simulink model "Digital-Memory-Architecture"  (R2024b)
settings: Solver=VariableStepAuto  StartTime=0.0  StopTime=10.0  RelTol=1e-3
libraries: simulink_extras x129
(part 2 of 5)

== system Digital-Memory-Architecture/8to1MUX7 ==
  Adress0 : Inport
  Adress1 : Inport  Port=2
  Adress2 : Inport  Port=3
  D0 : Inport  Port=4
  D1 : Inport  Port=5
  D2 : Inport  Port=6
  D3 : Inport  Port=7
  D4 : Inport  Port=8
  D5 : Inport  Port=9
  D6 : Inport  Port=10
  D7 : Inport  Port=11
  Logical Operator : Logic  Operator=NOT  IconShape=distinctive  AllPortsSameDT=off  OutDataTypeStr=boolean
  Logical Operator1 : Logic  Operator=NOT  IconShape=distinctive  AllPortsSameDT=off  OutDataTypeStr=boolean
  Logical Operator{4..11} (8 alike) : Logic  Inputs=4  IconShape=distinctive  AllPortsSameDT=off  OutDataTypeStr=boolean
  Logical Operator2 : Logic  Operator=NOT  IconShape=distinctive  AllPortsSameDT=off  OutDataTypeStr=boolean
  Logical Operator3 : Logic  Operator=OR  Inputs=8  IconShape=distinctive  AllPortsSameDT=off  OutDataTypeStr=boolean
  D : Outport
  wires:
  Logical Operator3/1 -> D/1
  Adress0/1 -> Logical Operator11/1, Logical Operator9/1, Logical Operator7/1, Logical Operator5/1, Logical Operator/1
  Adress1/1 -> Logical Operator11/2, Logical Operator10/2, Logical Operator7/2, Logical Operator6/2, Logical Operator1/1
  Adress2/1 -> Logical Operator11/3, Logical Operator10/3, Logical Operator9/3, Logical Operator8/3, Logical Operator2/1
  D7/1 -> Logical Operator11/4
  D6/1 -> Logical Operator10/4
  D5/1 -> Logical Operator9/4
  D4/1 -> Logical Operator8/4
  D3/1 -> Logical Operator7/4
  D2/1 -> Logical Operator6/4
  D1/1 -> Logical Operator5/4
  D0/1 -> Logical Operator4/4
  Logical Operator2/1 -> Logical Operator7/3, Logical Operator6/3, Logical Operator5/3, Logical Operator4/3
  Logical Operator1/1 -> Logical Operator9/2, Logical Operator8/2, Logical Operator5/2, Logical Operator4/2
  Logical Operator/1 -> Logical Operator10/1, Logical Operator8/1, Logical Operator6/1, Logical Operator4/1
  Logical Operator4/1 -> Logical Operator3/1
  Logical Operator5/1 -> Logical Operator3/2
  Logical Operator6/1 -> Logical Operator3/3
  Logical Operator7/1 -> Logical Operator3/4
  Logical Operator8/1 -> Logical Operator3/5
  Logical Operator9/1 -> Logical Operator3/6
  Logical Operator10/1 -> Logical Operator3/7
  Logical Operator11/1 -> Logical Operator3/8

== system Digital-Memory-Architecture/8to1MUX8 ==
  Adress0 : Inport
  Adress1 : Inport  Port=2
  Adress2 : Inport  Port=3
  D0 : Inport  Port=4
  D1 : Inport  Port=5
  D2 : Inport  Port=6
  D3 : Inport  Port=7
  D4 : Inport  Port=8
  D5 : Inport  Port=9
  D6 : Inport  Port=10
  D7 : Inport  Port=11
  Logical Operator : Logic  Operator=NOT  IconShape=distinctive  AllPortsSameDT=off  OutDataTypeStr=boolean
  Logical Operator1 : Logic  Operator=NOT  IconShape=distinctive  AllPortsSameDT=off  OutDataTypeStr=boolean
  Logical Operator{4..11} (8 alike) : Logic  Inputs=4  IconShape=distinctive  AllPortsSameDT=off  OutDataTypeStr=boolean
  Logical Operator2 : Logic  Operator=NOT  IconShape=distinctive  AllPortsSameDT=off  OutDataTypeStr=boolean
  Logical Operator3 : Logic  Operator=OR  Inputs=8  IconShape=distinctive  AllPortsSameDT=off  OutDataTypeStr=boolean
  A : Outport
  wires:
  Logical Operator3/1 -> A/1
  Adress0/1 -> Logical Operator11/1, Logical Operator9/1, Logical Operator7/1, Logical Operator5/1, Logical Operator/1
  Adress1/1 -> Logical Operator11/2, Logical Operator10/2, Logical Operator7/2, Logical Operator6/2, Logical Operator1/1
  Adress2/1 -> Logical Operator11/3, Logical Operator10/3, Logical Operator9/3, Logical Operator8/3, Logical Operator2/1
  D7/1 -> Logical Operator11/4
  D6/1 -> Logical Operator10/4
  D5/1 -> Logical Operator9/4
  D4/1 -> Logical Operator8/4
  D3/1 -> Logical Operator7/4
  D2/1 -> Logical Operator6/4
  D1/1 -> Logical Operator5/4
  D0/1 -> Logical Operator4/4
  Logical Operator2/1 -> Logical Operator7/3, Logical Operator6/3, Logical Operator5/3, Logical Operator4/3
  Logical Operator1/1 -> Logical Operator9/2, Logical Operator8/2, Logical Operator5/2, Logical Operator4/2
  Logical Operator/1 -> Logical Operator10/1, Logical Operator8/1, Logical Operator6/1, Logical Operator4/1
  Logical Operator4/1 -> Logical Operator3/1
  Logical Operator5/1 -> Logical Operator3/2
  Logical Operator6/1 -> Logical Operator3/3
  Logical Operator7/1 -> Logical Operator3/4
  Logical Operator8/1 -> Logical Operator3/5
  Logical Operator9/1 -> Logical Operator3/6
  Logical Operator10/1 -> Logical Operator3/7
  Logical Operator11/1 -> Logical Operator3/8

== system Digital-Memory-Architecture/8to1MUX9 ==
  Adress0 : Inport
  Adress1 : Inport  Port=2
  Adress2 : Inport  Port=3
  D0 : Inport  Port=4
  D1 : Inport  Port=5
  D2 : Inport  Port=6
  D3 : Inport  Port=7
  D4 : Inport  Port=8
  D5 : Inport  Port=9
  D6 : Inport  Port=10
  D7 : Inport  Port=11
  Logical Operator : Logic  Operator=NOT  IconShape=distinctive  AllPortsSameDT=off  OutDataTypeStr=boolean
  Logical Operator1 : Logic  Operator=NOT  IconShape=distinctive  AllPortsSameDT=off  OutDataTypeStr=boolean
  Logical Operator{4..11} (8 alike) : Logic  Inputs=4  IconShape=distinctive  AllPortsSameDT=off  OutDataTypeStr=boolean
  Logical Operator2 : Logic  Operator=NOT  IconShape=distinctive  AllPortsSameDT=off  OutDataTypeStr=boolean
  Logical Operator3 : Logic  Operator=OR  Inputs=8  IconShape=distinctive  AllPortsSameDT=off  OutDataTypeStr=boolean
  B : Outport
  wires:
  Logical Operator3/1 -> B/1
  Adress0/1 -> Logical Operator11/1, Logical Operator9/1, Logical Operator7/1, Logical Operator5/1, Logical Operator/1
  Adress1/1 -> Logical Operator11/2, Logical Operator10/2, Logical Operator7/2, Logical Operator6/2, Logical Operator1/1
  Adress2/1 -> Logical Operator11/3, Logical Operator10/3, Logical Operator9/3, Logical Operator8/3, Logical Operator2/1
  D7/1 -> Logical Operator11/4
  D6/1 -> Logical Operator10/4
  D5/1 -> Logical Operator9/4
  D4/1 -> Logical Operator8/4
  D3/1 -> Logical Operator7/4
  D2/1 -> Logical Operator6/4
  D1/1 -> Logical Operator5/4
  D0/1 -> Logical Operator4/4
  Logical Operator2/1 -> Logical Operator7/3, Logical Operator6/3, Logical Operator5/3, Logical Operator4/3
  Logical Operator1/1 -> Logical Operator9/2, Logical Operator8/2, Logical Operator5/2, Logical Operator4/2
  Logical Operator/1 -> Logical Operator10/1, Logical Operator8/1, Logical Operator6/1, Logical Operator4/1
  Logical Operator4/1 -> Logical Operator3/1
  Logical Operator5/1 -> Logical Operator3/2
  Logical Operator6/1 -> Logical Operator3/3
  Logical Operator7/1 -> Logical Operator3/4
  Logical Operator8/1 -> Logical Operator3/5
  Logical Operator9/1 -> Logical Operator3/6
  Logical Operator10/1 -> Logical Operator3/7
  Logical Operator11/1 -> Logical Operator3/8

== system Digital-Memory-Architecture/BitCell1 ==
  D : Inport
  WE : Inport  Port=2
  CLK : Inport  Port=3
  Constant : Constant
  D Flip-Flop : simulink_extras/Flip Flops/D Flip-Flop
  Logical Operator : Logic  Operator=NOT  IconShape=distinctive  AllPortsSameDT=off  OutDataTypeStr=boolean
  Logical Operator1 : Logic  IconShape=distinctive  AllPortsSameDT=off  OutDataTypeStr=boolean
  Logical Operator2 : Logic  IconShape=distinctive  AllPortsSameDT=off  OutDataTypeStr=boolean
  Logical Operator3 : Logic  Operator=OR  IconShape=distinctive  AllPortsSameDT=off  OutDataTypeStr=boolean
  Q : Outport
  wires:
  Logical Operator2/1 -> Logical Operator3/2
  CLK/1 -> D Flip-Flop/2
  Logical Operator1/1 -> Logical Operator3/1
  Constant/1 -> D Flip-Flop/3
  D Flip-Flop/1 -> Q/1, Logical Operator2/2
  Logical Operator3/1 -> D Flip-Flop/1
  Logical Operator/1 -> Logical Operator2/1
  WE/1 -> Logical Operator/1, Logical Operator1/2
  D/1 -> Logical Operator1/1

== system Digital-Memory-Architecture/BitCell10 ==
  D : Inport
  WE : Inport  Port=2
  CLK : Inport  Port=3
  Constant : Constant
  D Flip-Flop : simulink_extras/Flip Flops/D Flip-Flop
  Logical Operator : Logic  Operator=NOT  IconShape=distinctive  AllPortsSameDT=off  OutDataTypeStr=boolean
  Logical Operator1 : Logic  IconShape=distinctive  AllPortsSameDT=off  OutDataTypeStr=boolean
  Logical Operator2 : Logic  IconShape=distinctive  AllPortsSameDT=off  OutDataTypeStr=boolean
  Logical Operator3 : Logic  Operator=OR  IconShape=distinctive  AllPortsSameDT=off  OutDataTypeStr=boolean
  Q : Outport
  wires:
  Logical Operator2/1 -> Logical Operator3/2
  CLK/1 -> D Flip-Flop/2
  Logical Operator1/1 -> Logical Operator3/1
  Constant/1 -> D Flip-Flop/3
  D Flip-Flop/1 -> Q/1, Logical Operator2/2
  Logical Operator3/1 -> D Flip-Flop/1
  Logical Operator/1 -> Logical Operator2/1
  WE/1 -> Logical Operator/1, Logical Operator1/2
  D/1 -> Logical Operator1/1

== system Digital-Memory-Architecture/BitCell100 ==
  D : Inport
  WE : Inport  Port=2
  CLK : Inport  Port=3
  Constant : Constant
  D Flip-Flop : simulink_extras/Flip Flops/D Flip-Flop
  Logical Operator : Logic  Operator=NOT  IconShape=distinctive  AllPortsSameDT=off  OutDataTypeStr=boolean
  Logical Operator1 : Logic  IconShape=distinctive  AllPortsSameDT=off  OutDataTypeStr=boolean
  Logical Operator2 : Logic  IconShape=distinctive  AllPortsSameDT=off  OutDataTypeStr=boolean
  Logical Operator3 : Logic  Operator=OR  IconShape=distinctive  AllPortsSameDT=off  OutDataTypeStr=boolean
  Q : Outport
  wires:
  Logical Operator2/1 -> Logical Operator3/2
  CLK/1 -> D Flip-Flop/2
  Logical Operator1/1 -> Logical Operator3/1
  Constant/1 -> D Flip-Flop/3
  D Flip-Flop/1 -> Q/1, Logical Operator2/2
  Logical Operator3/1 -> D Flip-Flop/1
  Logical Operator/1 -> Logical Operator2/1
  WE/1 -> Logical Operator/1, Logical Operator1/2
  D/1 -> Logical Operator1/1

== system Digital-Memory-Architecture/BitCell101 ==
  D : Inport
  WE : Inport  Port=2
  CLK : Inport  Port=3
  Constant : Constant
  D Flip-Flop : simulink_extras/Flip Flops/D Flip-Flop
  Logical Operator : Logic  Operator=NOT  IconShape=distinctive  AllPortsSameDT=off  OutDataTypeStr=boolean
  Logical Operator1 : Logic  IconShape=distinctive  AllPortsSameDT=off  OutDataTypeStr=boolean
  Logical Operator2 : Logic  IconShape=distinctive  AllPortsSameDT=off  OutDataTypeStr=boolean
  Logical Operator3 : Logic  Operator=OR  IconShape=distinctive  AllPortsSameDT=off  OutDataTypeStr=boolean
  Q : Outport
  wires:
  Logical Operator2/1 -> Logical Operator3/2
  CLK/1 -> D Flip-Flop/2
  Logical Operator1/1 -> Logical Operator3/1
  Constant/1 -> D Flip-Flop/3
  D Flip-Flop/1 -> Q/1, Logical Operator2/2
  Logical Operator3/1 -> D Flip-Flop/1
  Logical Operator/1 -> Logical Operator2/1
  WE/1 -> Logical Operator/1, Logical Operator1/2
  D/1 -> Logical Operator1/1

== system Digital-Memory-Architecture/BitCell102 ==
  D : Inport
  WE : Inport  Port=2
  CLK : Inport  Port=3
  Constant : Constant
  D Flip-Flop : simulink_extras/Flip Flops/D Flip-Flop
  Logical Operator : Logic  Operator=NOT  IconShape=distinctive  AllPortsSameDT=off  OutDataTypeStr=boolean
  Logical Operator1 : Logic  IconShape=distinctive  AllPortsSameDT=off  OutDataTypeStr=boolean
  Logical Operator2 : Logic  IconShape=distinctive  AllPortsSameDT=off  OutDataTypeStr=boolean
  Logical Operator3 : Logic  Operator=OR  IconShape=distinctive  AllPortsSameDT=off  OutDataTypeStr=boolean
  Q : Outport
  wires:
  Logical Operator2/1 -> Logical Operator3/2
  CLK/1 -> D Flip-Flop/2
  Logical Operator1/1 -> Logical Operator3/1
  Constant/1 -> D Flip-Flop/3
  D Flip-Flop/1 -> Q/1, Logical Operator2/2
  Logical Operator3/1 -> D Flip-Flop/1
  Logical Operator/1 -> Logical Operator2/1
  WE/1 -> Logical Operator/1, Logical Operator1/2
  D/1 -> Logical Operator1/1

== system Digital-Memory-Architecture/BitCell103 ==
  D : Inport
  WE : Inport  Port=2
  CLK : Inport  Port=3
  Constant : Constant
  D Flip-Flop : simulink_extras/Flip Flops/D Flip-Flop
  Logical Operator : Logic  Operator=NOT  IconShape=distinctive  AllPortsSameDT=off  OutDataTypeStr=boolean
  Logical Operator1 : Logic  IconShape=distinctive  AllPortsSameDT=off  OutDataTypeStr=boolean
  Logical Operator2 : Logic  IconShape=distinctive  AllPortsSameDT=off  OutDataTypeStr=boolean
  Logical Operator3 : Logic  Operator=OR  IconShape=distinctive  AllPortsSameDT=off  OutDataTypeStr=boolean
  Q : Outport
  wires:
  Logical Operator2/1 -> Logical Operator3/2
  CLK/1 -> D Flip-Flop/2
  Logical Operator1/1 -> Logical Operator3/1
  Constant/1 -> D Flip-Flop/3
  D Flip-Flop/1 -> Q/1, Logical Operator2/2
  Logical Operator3/1 -> D Flip-Flop/1
  Logical Operator/1 -> Logical Operator2/1
  WE/1 -> Logical Operator/1, Logical Operator1/2
  D/1 -> Logical Operator1/1

== system Digital-Memory-Architecture/BitCell104 ==
  D : Inport
  WE : Inport  Port=2
  CLK : Inport  Port=3
  Constant : Constant
  D Flip-Flop : simulink_extras/Flip Flops/D Flip-Flop
  Logical Operator : Logic  Operator=NOT  IconShape=distinctive  AllPortsSameDT=off  OutDataTypeStr=boolean
  Logical Operator1 : Logic  IconShape=distinctive  AllPortsSameDT=off  OutDataTypeStr=boolean
  Logical Operator2 : Logic  IconShape=distinctive  AllPortsSameDT=off  OutDataTypeStr=boolean
  Logical Operator3 : Logic  Operator=OR  IconShape=distinctive  AllPortsSameDT=off  OutDataTypeStr=boolean
  Q : Outport
  wires:
  Logical Operator2/1 -> Logical Operator3/2
  CLK/1 -> D Flip-Flop/2
  Logical Operator1/1 -> Logical Operator3/1
  Constant/1 -> D Flip-Flop/3
  D Flip-Flop/1 -> Q/1, Logical Operator2/2
  Logical Operator3/1 -> D Flip-Flop/1
  Logical Operator/1 -> Logical Operator2/1
  WE/1 -> Logical Operator/1, Logical Operator1/2
  D/1 -> Logical Operator1/1

== system Digital-Memory-Architecture/BitCell105 ==
  D : Inport
  WE : Inport  Port=2
  CLK : Inport  Port=3
  Constant : Constant
  D Flip-Flop : simulink_extras/Flip Flops/D Flip-Flop
  Logical Operator : Logic  Operator=NOT  IconShape=distinctive  AllPortsSameDT=off  OutDataTypeStr=boolean
  Logical Operator1 : Logic  IconShape=distinctive  AllPortsSameDT=off  OutDataTypeStr=boolean
  Logical Operator2 : Logic  IconShape=distinctive  AllPortsSameDT=off  OutDataTypeStr=boolean
  Logical Operator3 : Logic  Operator=OR  IconShape=distinctive  AllPortsSameDT=off  OutDataTypeStr=boolean
  Q : Outport
  wires:
  Logical Operator2/1 -> Logical Operator3/2
  CLK/1 -> D Flip-Flop/2
  Logical Operator1/1 -> Logical Operator3/1
  Constant/1 -> D Flip-Flop/3
  D Flip-Flop/1 -> Q/1, Logical Operator2/2
  Logical Operator3/1 -> D Flip-Flop/1
  Logical Operator/1 -> Logical Operator2/1
  WE/1 -> Logical Operator/1, Logical Operator1/2
  D/1 -> Logical Operator1/1

== system Digital-Memory-Architecture/BitCell106 ==
  D : Inport
  WE : Inport  Port=2
  CLK : Inport  Port=3
  Constant : Constant
  D Flip-Flop : simulink_extras/Flip Flops/D Flip-Flop
  Logical Operator : Logic  Operator=NOT  IconShape=distinctive  AllPortsSameDT=off  OutDataTypeStr=boolean
  Logical Operator1 : Logic  IconShape=distinctive  AllPortsSameDT=off  OutDataTypeStr=boolean
  Logical Operator2 : Logic  IconShape=distinctive  AllPortsSameDT=off  OutDataTypeStr=boolean
  Logical Operator3 : Logic  Operator=OR  IconShape=distinctive  AllPortsSameDT=off  OutDataTypeStr=boolean
  Q : Outport
  wires:
  Logical Operator2/1 -> Logical Operator3/2
  CLK/1 -> D Flip-Flop/2
  Logical Operator1/1 -> Logical Operator3/1
  Constant/1 -> D Flip-Flop/3
  D Flip-Flop/1 -> Q/1, Logical Operator2/2
  Logical Operator3/1 -> D Flip-Flop/1
  Logical Operator/1 -> Logical Operator2/1
  WE/1 -> Logical Operator/1, Logical Operator1/2
  D/1 -> Logical Operator1/1

== system Digital-Memory-Architecture/BitCell107 ==
  D : Inport
  WE : Inport  Port=2
  CLK : Inport  Port=3
  Constant : Constant
  D Flip-Flop : simulink_extras/Flip Flops/D Flip-Flop
  Logical Operator : Logic  Operator=NOT  IconShape=distinctive  AllPortsSameDT=off  OutDataTypeStr=boolean
  Logical Operator1 : Logic  IconShape=distinctive  AllPortsSameDT=off  OutDataTypeStr=boolean
  Logical Operator2 : Logic  IconShape=distinctive  AllPortsSameDT=off  OutDataTypeStr=boolean
  Logical Operator3 : Logic  Operator=OR  IconShape=distinctive  AllPortsSameDT=off  OutDataTypeStr=boolean
  Q : Outport
  wires:
  Logical Operator2/1 -> Logical Operator3/2
  CLK/1 -> D Flip-Flop/2
  Logical Operator1/1 -> Logical Operator3/1
  Constant/1 -> D Flip-Flop/3
  D Flip-Flop/1 -> Q/1, Logical Operator2/2
  Logical Operator3/1 -> D Flip-Flop/1
  Logical Operator/1 -> Logical Operator2/1
  WE/1 -> Logical Operator/1, Logical Operator1/2
  D/1 -> Logical Operator1/1

== system Digital-Memory-Architecture/BitCell108 ==
  D : Inport
  WE : Inport  Port=2
  CLK : Inport  Port=3
  Constant : Constant
  D Flip-Flop : simulink_extras/Flip Flops/D Flip-Flop
  Logical Operator : Logic  Operator=NOT  IconShape=distinctive  AllPortsSameDT=off  OutDataTypeStr=boolean
  Logical Operator1 : Logic  IconShape=distinctive  AllPortsSameDT=off  OutDataTypeStr=boolean
  Logical Operator2 : Logic  IconShape=distinctive  AllPortsSameDT=off  OutDataTypeStr=boolean
  Logical Operator3 : Logic  Operator=OR  IconShape=distinctive  AllPortsSameDT=off  OutDataTypeStr=boolean
  Q : Outport
  wires:
  Logical Operator2/1 -> Logical Operator3/2
  CLK/1 -> D Flip-Flop/2
  Logical Operator1/1 -> Logical Operator3/1
  Constant/1 -> D Flip-Flop/3
  D Flip-Flop/1 -> Q/1, Logical Operator2/2
  Logical Operator3/1 -> D Flip-Flop/1
  Logical Operator/1 -> Logical Operator2/1
  WE/1 -> Logical Operator/1, Logical Operator1/2
  D/1 -> Logical Operator1/1

== system Digital-Memory-Architecture/BitCell109 ==
  D : Inport
  WE : Inport  Port=2
  CLK : Inport  Port=3
  Constant : Constant
  D Flip-Flop : simulink_extras/Flip Flops/D Flip-Flop
  Logical Operator : Logic  Operator=NOT  IconShape=distinctive  AllPortsSameDT=off  OutDataTypeStr=boolean
  Logical Operator1 : Logic  IconShape=distinctive  AllPortsSameDT=off  OutDataTypeStr=boolean
  Logical Operator2 : Logic  IconShape=distinctive  AllPortsSameDT=off  OutDataTypeStr=boolean
  Logical Operator3 : Logic  Operator=OR  IconShape=distinctive  AllPortsSameDT=off  OutDataTypeStr=boolean
  Q : Outport
  wires:
  Logical Operator2/1 -> Logical Operator3/2
  CLK/1 -> D Flip-Flop/2
  Logical Operator1/1 -> Logical Operator3/1
  Constant/1 -> D Flip-Flop/3
  D Flip-Flop/1 -> Q/1, Logical Operator2/2
  Logical Operator3/1 -> D Flip-Flop/1
  Logical Operator/1 -> Logical Operator2/1
  WE/1 -> Logical Operator/1, Logical Operator1/2
  D/1 -> Logical Operator1/1

== system Digital-Memory-Architecture/BitCell11 ==
  D : Inport
  WE : Inport  Port=2
  CLK : Inport  Port=3
  Constant : Constant
  D Flip-Flop : simulink_extras/Flip Flops/D Flip-Flop
  Logical Operator : Logic  Operator=NOT  IconShape=distinctive  AllPortsSameDT=off  OutDataTypeStr=boolean
  Logical Operator1 : Logic  IconShape=distinctive  AllPortsSameDT=off  OutDataTypeStr=boolean
  Logical Operator2 : Logic  IconShape=distinctive  AllPortsSameDT=off  OutDataTypeStr=boolean
  Logical Operator3 : Logic  Operator=OR  IconShape=distinctive  AllPortsSameDT=off  OutDataTypeStr=boolean
  Q : Outport
  wires:
  Logical Operator2/1 -> Logical Operator3/2
  CLK/1 -> D Flip-Flop/2
  Logical Operator1/1 -> Logical Operator3/1
  Constant/1 -> D Flip-Flop/3
  D Flip-Flop/1 -> Q/1, Logical Operator2/2
  Logical Operator3/1 -> D Flip-Flop/1
  Logical Operator/1 -> Logical Operator2/1
  WE/1 -> Logical Operator/1, Logical Operator1/2
  D/1 -> Logical Operator1/1

== system Digital-Memory-Architecture/BitCell110 ==
  D : Inport
  WE : Inport  Port=2
  CLK : Inport  Port=3
  Constant : Constant
  D Flip-Flop : simulink_extras/Flip Flops/D Flip-Flop
  Logical Operator : Logic  Operator=NOT  IconShape=distinctive  AllPortsSameDT=off  OutDataTypeStr=boolean
  Logical Operator1 : Logic  IconShape=distinctive  AllPortsSameDT=off  OutDataTypeStr=boolean
  Logical Operator2 : Logic  IconShape=distinctive  AllPortsSameDT=off  OutDataTypeStr=boolean
  Logical Operator3 : Logic  Operator=OR  IconShape=distinctive  AllPortsSameDT=off  OutDataTypeStr=boolean
  Q : Outport
  wires:
  Logical Operator2/1 -> Logical Operator3/2
  CLK/1 -> D Flip-Flop/2
  Logical Operator1/1 -> Logical Operator3/1
  Constant/1 -> D Flip-Flop/3
  D Flip-Flop/1 -> Q/1, Logical Operator2/2
  Logical Operator3/1 -> D Flip-Flop/1
  Logical Operator/1 -> Logical Operator2/1
  WE/1 -> Logical Operator/1, Logical Operator1/2
  D/1 -> Logical Operator1/1

== system Digital-Memory-Architecture/BitCell111 ==
  D : Inport
  WE : Inport  Port=2
  CLK : Inport  Port=3
  Constant : Constant
  D Flip-Flop : simulink_extras/Flip Flops/D Flip-Flop
  Logical Operator : Logic  Operator=NOT  IconShape=distinctive  AllPortsSameDT=off  OutDataTypeStr=boolean
  Logical Operator1 : Logic  IconShape=distinctive  AllPortsSameDT=off  OutDataTypeStr=boolean
  Logical Operator2 : Logic  IconShape=distinctive  AllPortsSameDT=off  OutDataTypeStr=boolean
  Logical Operator3 : Logic  Operator=OR  IconShape=distinctive  AllPortsSameDT=off  OutDataTypeStr=boolean
  Q : Outport
  wires:
  Logical Operator2/1 -> Logical Operator3/2
  CLK/1 -> D Flip-Flop/2
  Logical Operator1/1 -> Logical Operator3/1
  Constant/1 -> D Flip-Flop/3
  D Flip-Flop/1 -> Q/1, Logical Operator2/2
  Logical Operator3/1 -> D Flip-Flop/1
  Logical Operator/1 -> Logical Operator2/1
  WE/1 -> Logical Operator/1, Logical Operator1/2
  D/1 -> Logical Operator1/1

== system Digital-Memory-Architecture/BitCell112 ==
  D : Inport
  WE : Inport  Port=2
  CLK : Inport  Port=3
  Constant : Constant
  D Flip-Flop : simulink_extras/Flip Flops/D Flip-Flop
  Logical Operator : Logic  Operator=NOT  IconShape=distinctive  AllPortsSameDT=off  OutDataTypeStr=boolean
  Logical Operator1 : Logic  IconShape=distinctive  AllPortsSameDT=off  OutDataTypeStr=boolean
  Logical Operator2 : Logic  IconShape=distinctive  AllPortsSameDT=off  OutDataTypeStr=boolean
  Logical Operator3 : Logic  Operator=OR  IconShape=distinctive  AllPortsSameDT=off  OutDataTypeStr=boolean
  Q : Outport
  wires:
  Logical Operator2/1 -> Logical Operator3/2
  CLK/1 -> D Flip-Flop/2
  Logical Operator1/1 -> Logical Operator3/1
  Constant/1 -> D Flip-Flop/3
  D Flip-Flop/1 -> Q/1, Logical Operator2/2
  Logical Operator3/1 -> D Flip-Flop/1
  Logical Operator/1 -> Logical Operator2/1
  WE/1 -> Logical Operator/1, Logical Operator1/2
  D/1 -> Logical Operator1/1

== system Digital-Memory-Architecture/BitCell113 ==
  D : Inport
  WE : Inport  Port=2
  CLK : Inport  Port=3
  Constant : Constant
  D Flip-Flop : simulink_extras/Flip Flops/D Flip-Flop
  Logical Operator : Logic  Operator=NOT  IconShape=distinctive  AllPortsSameDT=off  OutDataTypeStr=boolean
  Logical Operator1 : Logic  IconShape=distinctive  AllPortsSameDT=off  OutDataTypeStr=boolean
  Logical Operator2 : Logic  IconShape=distinctive  AllPortsSameDT=off  OutDataTypeStr=boolean
  Logical Operator3 : Logic  Operator=OR  IconShape=distinctive  AllPortsSameDT=off  OutDataTypeStr=boolean
  Q : Outport
  wires:
  Logical Operator2/1 -> Logical Operator3/2
  CLK/1 -> D Flip-Flop/2
  Logical Operator1/1 -> Logical Operator3/1
  Constant/1 -> D Flip-Flop/3
  D Flip-Flop/1 -> Q/1, Logical Operator2/2
  Logical Operator3/1 -> D Flip-Flop/1
  Logical Operator/1 -> Logical Operator2/1
  WE/1 -> Logical Operator/1, Logical Operator1/2
  D/1 -> Logical Operator1/1

== system Digital-Memory-Architecture/BitCell114 ==
  D : Inport
  WE : Inport  Port=2
  CLK : Inport  Port=3
  Constant : Constant
  D Flip-Flop : simulink_extras/Flip Flops/D Flip-Flop
  Logical Operator : Logic  Operator=NOT  IconShape=distinctive  AllPortsSameDT=off  OutDataTypeStr=boolean
  Logical Operator1 : Logic  IconShape=distinctive  AllPortsSameDT=off  OutDataTypeStr=boolean
  Logical Operator2 : Logic  IconShape=distinctive  AllPortsSameDT=off  OutDataTypeStr=boolean
  Logical Operator3 : Logic  Operator=OR  IconShape=distinctive  AllPortsSameDT=off  OutDataTypeStr=boolean
  Q : Outport
  wires:
  Logical Operator2/1 -> Logical Operator3/2
  CLK/1 -> D Flip-Flop/2
  Logical Operator1/1 -> Logical Operator3/1
  Constant/1 -> D Flip-Flop/3
  D Flip-Flop/1 -> Q/1, Logical Operator2/2
  Logical Operator3/1 -> D Flip-Flop/1
  Logical Operator/1 -> Logical Operator2/1
  WE/1 -> Logical Operator/1, Logical Operator1/2
  D/1 -> Logical Operator1/1

== system Digital-Memory-Architecture/BitCell115 ==
  D : Inport
  WE : Inport  Port=2
  CLK : Inport  Port=3
  Constant : Constant
  D Flip-Flop : simulink_extras/Flip Flops/D Flip-Flop
  Logical Operator : Logic  Operator=NOT  IconShape=distinctive  AllPortsSameDT=off  OutDataTypeStr=boolean
  Logical Operator1 : Logic  IconShape=distinctive  AllPortsSameDT=off  OutDataTypeStr=boolean
  Logical Operator2 : Logic  IconShape=distinctive  AllPortsSameDT=off  OutDataTypeStr=boolean
  Logical Operator3 : Logic  Operator=OR  IconShape=distinctive  AllPortsSameDT=off  OutDataTypeStr=boolean
  Q : Outport
  wires:
  Logical Operator2/1 -> Logical Operator3/2
  CLK/1 -> D Flip-Flop/2
  Logical Operator1/1 -> Logical Operator3/1
  Constant/1 -> D Flip-Flop/3
  D Flip-Flop/1 -> Q/1, Logical Operator2/2
  Logical Operator3/1 -> D Flip-Flop/1
  Logical Operator/1 -> Logical Operator2/1
  WE/1 -> Logical Operator/1, Logical Operator1/2
  D/1 -> Logical Operator1/1

== system Digital-Memory-Architecture/BitCell116 ==
  D : Inport
  WE : Inport  Port=2
  CLK : Inport  Port=3
  Constant : Constant
  D Flip-Flop : simulink_extras/Flip Flops/D Flip-Flop
  Logical Operator : Logic  Operator=NOT  IconShape=distinctive  AllPortsSameDT=off  OutDataTypeStr=boolean
  Logical Operator1 : Logic  IconShape=distinctive  AllPortsSameDT=off  OutDataTypeStr=boolean
  Logical Operator2 : Logic  IconShape=distinctive  AllPortsSameDT=off  OutDataTypeStr=boolean
  Logical Operator3 : Logic  Operator=OR  IconShape=distinctive  AllPortsSameDT=off  OutDataTypeStr=boolean
  Q : Outport
  wires:
  Logical Operator2/1 -> Logical Operator3/2
  CLK/1 -> D Flip-Flop/2
  Logical Operator1/1 -> Logical Operator3/1
  Constant/1 -> D Flip-Flop/3
  D Flip-Flop/1 -> Q/1, Logical Operator2/2
  Logical Operator3/1 -> D Flip-Flop/1
  Logical Operator/1 -> Logical Operator2/1
  WE/1 -> Logical Operator/1, Logical Operator1/2
  D/1 -> Logical Operator1/1

== system Digital-Memory-Architecture/BitCell117 ==
  D : Inport
  WE : Inport  Port=2
  CLK : Inport  Port=3
  Constant : Constant
  D Flip-Flop : simulink_extras/Flip Flops/D Flip-Flop
  Logical Operator : Logic  Operator=NOT  IconShape=distinctive  AllPortsSameDT=off  OutDataTypeStr=boolean
  Logical Operator1 : Logic  IconShape=distinctive  AllPortsSameDT=off  OutDataTypeStr=boolean
  Logical Operator2 : Logic  IconShape=distinctive  AllPortsSameDT=off  OutDataTypeStr=boolean
  Logical Operator3 : Logic  Operator=OR  IconShape=distinctive  AllPortsSameDT=off  OutDataTypeStr=boolean
  Q : Outport
  wires:
  Logical Operator2/1 -> Logical Operator3/2
  CLK/1 -> D Flip-Flop/2
  Logical Operator1/1 -> Logical Operator3/1
  Constant/1 -> D Flip-Flop/3
  D Flip-Flop/1 -> Q/1, Logical Operator2/2
  Logical Operator3/1 -> D Flip-Flop/1
  Logical Operator/1 -> Logical Operator2/1
  WE/1 -> Logical Operator/1, Logical Operator1/2
  D/1 -> Logical Operator1/1

== system Digital-Memory-Architecture/BitCell118 ==
  D : Inport
  WE : Inport  Port=2
  CLK : Inport  Port=3
  Constant : Constant
  D Flip-Flop : simulink_extras/Flip Flops/D Flip-Flop
  Logical Operator : Logic  Operator=NOT  IconShape=distinctive  AllPortsSameDT=off  OutDataTypeStr=boolean
  Logical Operator1 : Logic  IconShape=distinctive  AllPortsSameDT=off  OutDataTypeStr=boolean
  Logical Operator2 : Logic  IconShape=distinctive  AllPortsSameDT=off  OutDataTypeStr=boolean
  Logical Operator3 : Logic  Operator=OR  IconShape=distinctive  AllPortsSameDT=off  OutDataTypeStr=boolean
  Q : Outport
  wires:
  Logical Operator2/1 -> Logical Operator3/2
  CLK/1 -> D Flip-Flop/2
  Logical Operator1/1 -> Logical Operator3/1
  Constant/1 -> D Flip-Flop/3
  D Flip-Flop/1 -> Q/1, Logical Operator2/2
  Logical Operator3/1 -> D Flip-Flop/1
  Logical Operator/1 -> Logical Operator2/1
  WE/1 -> Logical Operator/1, Logical Operator1/2
  D/1 -> Logical Operator1/1

== system Digital-Memory-Architecture/BitCell119 ==
  D : Inport
  WE : Inport  Port=2
  CLK : Inport  Port=3
  Constant : Constant
  D Flip-Flop : simulink_extras/Flip Flops/D Flip-Flop
  Logical Operator : Logic  Operator=NOT  IconShape=distinctive  AllPortsSameDT=off  OutDataTypeStr=boolean
  Logical Operator1 : Logic  IconShape=distinctive  AllPortsSameDT=off  OutDataTypeStr=boolean
  Logical Operator2 : Logic  IconShape=distinctive  AllPortsSameDT=off  OutDataTypeStr=boolean
  Logical Operator3 : Logic  Operator=OR  IconShape=distinctive  AllPortsSameDT=off  OutDataTypeStr=boolean
  Q : Outport
  wires:
  Logical Operator2/1 -> Logical Operator3/2
  CLK/1 -> D Flip-Flop/2
  Logical Operator1/1 -> Logical Operator3/1
  Constant/1 -> D Flip-Flop/3
  D Flip-Flop/1 -> Q/1, Logical Operator2/2
  Logical Operator3/1 -> D Flip-Flop/1
  Logical Operator/1 -> Logical Operator2/1
  WE/1 -> Logical Operator/1, Logical Operator1/2
  D/1 -> Logical Operator1/1

== system Digital-Memory-Architecture/BitCell12 ==
  D : Inport
  WE : Inport  Port=2
  CLK : Inport  Port=3
  Constant : Constant
  D Flip-Flop : simulink_extras/Flip Flops/D Flip-Flop
  Logical Operator : Logic  Operator=NOT  IconShape=distinctive  AllPortsSameDT=off  OutDataTypeStr=boolean
  Logical Operator1 : Logic  IconShape=distinctive  AllPortsSameDT=off  OutDataTypeStr=boolean
  Logical Operator2 : Logic  IconShape=distinctive  AllPortsSameDT=off  OutDataTypeStr=boolean
  Logical Operator3 : Logic  Operator=OR  IconShape=distinctive  AllPortsSameDT=off  OutDataTypeStr=boolean
  Q : Outport
  wires:
  Logical Operator2/1 -> Logical Operator3/2
  CLK/1 -> D Flip-Flop/2
  Logical Operator1/1 -> Logical Operator3/1
  Constant/1 -> D Flip-Flop/3
  D Flip-Flop/1 -> Q/1, Logical Operator2/2
  Logical Operator3/1 -> D Flip-Flop/1
  Logical Operator/1 -> Logical Operator2/1
  WE/1 -> Logical Operator/1, Logical Operator1/2
  D/1 -> Logical Operator1/1

== system Digital-Memory-Architecture/BitCell120 ==
  D : Inport
  WE : Inport  Port=2
  CLK : Inport  Port=3
  Constant : Constant
  D Flip-Flop : simulink_extras/Flip Flops/D Flip-Flop
  Logical Operator : Logic  Operator=NOT  IconShape=distinctive  AllPortsSameDT=off  OutDataTypeStr=boolean
  Logical Operator1 : Logic  IconShape=distinctive  AllPortsSameDT=off  OutDataTypeStr=boolean
  Logical Operator2 : Logic  IconShape=distinctive  AllPortsSameDT=off  OutDataTypeStr=boolean
  Logical Operator3 : Logic  Operator=OR  IconShape=distinctive  AllPortsSameDT=off  OutDataTypeStr=boolean
  Q : Outport
  wires:
  Logical Operator2/1 -> Logical Operator3/2
  CLK/1 -> D Flip-Flop/2
  Logical Operator1/1 -> Logical Operator3/1
  Constant/1 -> D Flip-Flop/3
  D Flip-Flop/1 -> Q/1, Logical Operator2/2
  Logical Operator3/1 -> D Flip-Flop/1
  Logical Operator/1 -> Logical Operator2/1
  WE/1 -> Logical Operator/1, Logical Operator1/2
  D/1 -> Logical Operator1/1

== system Digital-Memory-Architecture/BitCell121 ==
  D : Inport
  WE : Inport  Port=2
  CLK : Inport  Port=3
  Constant : Constant
  D Flip-Flop : simulink_extras/Flip Flops/D Flip-Flop
  Logical Operator : Logic  Operator=NOT  IconShape=distinctive  AllPortsSameDT=off  OutDataTypeStr=boolean
  Logical Operator1 : Logic  IconShape=distinctive  AllPortsSameDT=off  OutDataTypeStr=boolean
  Logical Operator2 : Logic  IconShape=distinctive  AllPortsSameDT=off  OutDataTypeStr=boolean
  Logical Operator3 : Logic  Operator=OR  IconShape=distinctive  AllPortsSameDT=off  OutDataTypeStr=boolean
  Q : Outport
  wires:
  Logical Operator2/1 -> Logical Operator3/2
  CLK/1 -> D Flip-Flop/2
  Logical Operator1/1 -> Logical Operator3/1
  Constant/1 -> D Flip-Flop/3
  D Flip-Flop/1 -> Q/1, Logical Operator2/2
  Logical Operator3/1 -> D Flip-Flop/1
  Logical Operator/1 -> Logical Operator2/1
  WE/1 -> Logical Operator/1, Logical Operator1/2
  D/1 -> Logical Operator1/1

== system Digital-Memory-Architecture/BitCell122 ==
  D : Inport
  WE : Inport  Port=2
  CLK : Inport  Port=3
  Constant : Constant
  D Flip-Flop : simulink_extras/Flip Flops/D Flip-Flop
  Logical Operator : Logic  Operator=NOT  IconShape=distinctive  AllPortsSameDT=off  OutDataTypeStr=boolean
  Logical Operator1 : Logic  IconShape=distinctive  AllPortsSameDT=off  OutDataTypeStr=boolean
  Logical Operator2 : Logic  IconShape=distinctive  AllPortsSameDT=off  OutDataTypeStr=boolean
  Logical Operator3 : Logic  Operator=OR  IconShape=distinctive  AllPortsSameDT=off  OutDataTypeStr=boolean
  Q : Outport
  wires:
  Logical Operator2/1 -> Logical Operator3/2
  CLK/1 -> D Flip-Flop/2
  Logical Operator1/1 -> Logical Operator3/1
  Constant/1 -> D Flip-Flop/3
  D Flip-Flop/1 -> Q/1, Logical Operator2/2
  Logical Operator3/1 -> D Flip-Flop/1
  Logical Operator/1 -> Logical Operator2/1
  WE/1 -> Logical Operator/1, Logical Operator1/2
  D/1 -> Logical Operator1/1

== system Digital-Memory-Architecture/BitCell123 ==
  D : Inport
  WE : Inport  Port=2
  CLK : Inport  Port=3
  Constant : Constant
  D Flip-Flop : simulink_extras/Flip Flops/D Flip-Flop
  Logical Operator : Logic  Operator=NOT  IconShape=distinctive  AllPortsSameDT=off  OutDataTypeStr=boolean
  Logical Operator1 : Logic  IconShape=distinctive  AllPortsSameDT=off  OutDataTypeStr=boolean
  Logical Operator2 : Logic  IconShape=distinctive  AllPortsSameDT=off  OutDataTypeStr=boolean
  Logical Operator3 : Logic  Operator=OR  IconShape=distinctive  AllPortsSameDT=off  OutDataTypeStr=boolean
  Q : Outport
  wires:
  Logical Operator2/1 -> Logical Operator3/2
  CLK/1 -> D Flip-Flop/2
  Logical Operator1/1 -> Logical Operator3/1
  Constant/1 -> D Flip-Flop/3
  D Flip-Flop/1 -> Q/1, Logical Operator2/2
  Logical Operator3/1 -> D Flip-Flop/1
  Logical Operator/1 -> Logical Operator2/1
  WE/1 -> Logical Operator/1, Logical Operator1/2
  D/1 -> Logical Operator1/1

== system Digital-Memory-Architecture/BitCell124 ==
  D : Inport
  WE : Inport  Port=2
  CLK : Inport  Port=3
  Constant : Constant
  D Flip-Flop : simulink_extras/Flip Flops/D Flip-Flop
  Logical Operator : Logic  Operator=NOT  IconShape=distinctive  AllPortsSameDT=off  OutDataTypeStr=boolean
  Logical Operator1 : Logic  IconShape=distinctive  AllPortsSameDT=off  OutDataTypeStr=boolean
  Logical Operator2 : Logic  IconShape=distinctive  AllPortsSameDT=off  OutDataTypeStr=boolean
  Logical Operator3 : Logic  Operator=OR  IconShape=distinctive  AllPortsSameDT=off  OutDataTypeStr=boolean
  Q : Outport
  wires:
  Logical Operator2/1 -> Logical Operator3/2
  CLK/1 -> D Flip-Flop/2
  Logical Operator1/1 -> Logical Operator3/1
  Constant/1 -> D Flip-Flop/3
  D Flip-Flop/1 -> Q/1, Logical Operator2/2
  Logical Operator3/1 -> D Flip-Flop/1
  Logical Operator/1 -> Logical Operator2/1
  WE/1 -> Logical Operator/1, Logical Operator1/2
  D/1 -> Logical Operator1/1

== system Digital-Memory-Architecture/BitCell125 ==
  D : Inport
  WE : Inport  Port=2
  CLK : Inport  Port=3
  Constant : Constant
  D Flip-Flop : simulink_extras/Flip Flops/D Flip-Flop
  Logical Operator : Logic  Operator=NOT  IconShape=distinctive  AllPortsSameDT=off  OutDataTypeStr=boolean
  Logical Operator1 : Logic  IconShape=distinctive  AllPortsSameDT=off  OutDataTypeStr=boolean
  Logical Operator2 : Logic  IconShape=distinctive  AllPortsSameDT=off  OutDataTypeStr=boolean
  Logical Operator3 : Logic  Operator=OR  IconShape=distinctive  AllPortsSameDT=off  OutDataTypeStr=boolean
  Q : Outport
  wires:
  Logical Operator2/1 -> Logical Operator3/2
  CLK/1 -> D Flip-Flop/2
  Logical Operator1/1 -> Logical Operator3/1
  Constant/1 -> D Flip-Flop/3
  D Flip-Flop/1 -> Q/1, Logical Operator2/2
  Logical Operator3/1 -> D Flip-Flop/1
  Logical Operator/1 -> Logical Operator2/1
  WE/1 -> Logical Operator/1, Logical Operator1/2
  D/1 -> Logical Operator1/1

== system Digital-Memory-Architecture/BitCell126 ==
  D : Inport
  WE : Inport  Port=2
  CLK : Inport  Port=3
  Constant : Constant
  D Flip-Flop : simulink_extras/Flip Flops/D Flip-Flop
  Logical Operator : Logic  Operator=NOT  IconShape=distinctive  AllPortsSameDT=off  OutDataTypeStr=boolean
  Logical Operator1 : Logic  IconShape=distinctive  AllPortsSameDT=off  OutDataTypeStr=boolean
  Logical Operator2 : Logic  IconShape=distinctive  AllPortsSameDT=off  OutDataTypeStr=boolean
  Logical Operator3 : Logic  Operator=OR  IconShape=distinctive  AllPortsSameDT=off  OutDataTypeStr=boolean
  Q : Outport
  wires:
  Logical Operator2/1 -> Logical Operator3/2
  CLK/1 -> D Flip-Flop/2
  Logical Operator1/1 -> Logical Operator3/1
  Constant/1 -> D Flip-Flop/3
  D Flip-Flop/1 -> Q/1, Logical Operator2/2
  Logical Operator3/1 -> D Flip-Flop/1
  Logical Operator/1 -> Logical Operator2/1
  WE/1 -> Logical Operator/1, Logical Operator1/2
  D/1 -> Logical Operator1/1

== system Digital-Memory-Architecture/BitCell127 ==
  D : Inport
  WE : Inport  Port=2
  CLK : Inport  Port=3
  Constant : Constant
  D Flip-Flop : simulink_extras/Flip Flops/D Flip-Flop
  Logical Operator : Logic  Operator=NOT  IconShape=distinctive  AllPortsSameDT=off  OutDataTypeStr=boolean
  Logical Operator1 : Logic  IconShape=distinctive  AllPortsSameDT=off  OutDataTypeStr=boolean
  Logical Operator2 : Logic  IconShape=distinctive  AllPortsSameDT=off  OutDataTypeStr=boolean
  Logical Operator3 : Logic  Operator=OR  IconShape=distinctive  AllPortsSameDT=off  OutDataTypeStr=boolean
  Q : Outport
  wires:
  Logical Operator2/1 -> Logical Operator3/2
  CLK/1 -> D Flip-Flop/2
  Logical Operator1/1 -> Logical Operator3/1
  Constant/1 -> D Flip-Flop/3
  D Flip-Flop/1 -> Q/1, Logical Operator2/2
  Logical Operator3/1 -> D Flip-Flop/1
  Logical Operator/1 -> Logical Operator2/1
  WE/1 -> Logical Operator/1, Logical Operator1/2
  D/1 -> Logical Operator1/1

== system Digital-Memory-Architecture/BitCell128 ==
  D : Inport
  WE : Inport  Port=2
  CLK : Inport  Port=3
  Constant : Constant
  D Flip-Flop : simulink_extras/Flip Flops/D Flip-Flop
  Logical Operator : Logic  Operator=NOT  IconShape=distinctive  AllPortsSameDT=off  OutDataTypeStr=boolean
  Logical Operator1 : Logic  IconShape=distinctive  AllPortsSameDT=off  OutDataTypeStr=boolean
  Logical Operator2 : Logic  IconShape=distinctive  AllPortsSameDT=off  OutDataTypeStr=boolean
  Logical Operator3 : Logic  Operator=OR  IconShape=distinctive  AllPortsSameDT=off  OutDataTypeStr=boolean
  Q : Outport
  wires:
  Logical Operator2/1 -> Logical Operator3/2
  CLK/1 -> D Flip-Flop/2
  Logical Operator1/1 -> Logical Operator3/1
  Constant/1 -> D Flip-Flop/3
  D Flip-Flop/1 -> Q/1, Logical Operator2/2
  Logical Operator3/1 -> D Flip-Flop/1
  Logical Operator/1 -> Logical Operator2/1
  WE/1 -> Logical Operator/1, Logical Operator1/2
  D/1 -> Logical Operator1/1

== system Digital-Memory-Architecture/BitCell13 ==
  D : Inport
  WE : Inport  Port=2
  CLK : Inport  Port=3
  Constant : Constant
  D Flip-Flop : simulink_extras/Flip Flops/D Flip-Flop
  Logical Operator : Logic  Operator=NOT  IconShape=distinctive  AllPortsSameDT=off  OutDataTypeStr=boolean
  Logical Operator1 : Logic  IconShape=distinctive  AllPortsSameDT=off  OutDataTypeStr=boolean
  Logical Operator2 : Logic  IconShape=distinctive  AllPortsSameDT=off  OutDataTypeStr=boolean
  Logical Operator3 : Logic  Operator=OR  IconShape=distinctive  AllPortsSameDT=off  OutDataTypeStr=boolean
  Q : Outport
  wires:
  Logical Operator2/1 -> Logical Operator3/2
  CLK/1 -> D Flip-Flop/2
  Logical Operator1/1 -> Logical Operator3/1
  Constant/1 -> D Flip-Flop/3
  D Flip-Flop/1 -> Q/1, Logical Operator2/2
  Logical Operator3/1 -> D Flip-Flop/1
  Logical Operator/1 -> Logical Operator2/1
  WE/1 -> Logical Operator/1, Logical Operator1/2
  D/1 -> Logical Operator1/1

== system Digital-Memory-Architecture/BitCell14 ==
  D : Inport
  WE : Inport  Port=2
  CLK : Inport  Port=3
  Constant : Constant
  D Flip-Flop : simulink_extras/Flip Flops/D Flip-Flop
  Logical Operator : Logic  Operator=NOT  IconShape=distinctive  AllPortsSameDT=off  OutDataTypeStr=boolean
  Logical Operator1 : Logic  IconShape=distinctive  AllPortsSameDT=off  OutDataTypeStr=boolean
  Logical Operator2 : Logic  IconShape=distinctive  AllPortsSameDT=off  OutDataTypeStr=boolean
  Logical Operator3 : Logic  Operator=OR  IconShape=distinctive  AllPortsSameDT=off  OutDataTypeStr=boolean
  Q : Outport
  wires:
  Logical Operator2/1 -> Logical Operator3/2
  CLK/1 -> D Flip-Flop/2
  Logical Operator1/1 -> Logical Operator3/1
  Constant/1 -> D Flip-Flop/3
  D Flip-Flop/1 -> Q/1, Logical Operator2/2
  Logical Operator3/1 -> D Flip-Flop/1
  Logical Operator/1 -> Logical Operator2/1
  WE/1 -> Logical Operator/1, Logical Operator1/2
  D/1 -> Logical Operator1/1

== system Digital-Memory-Architecture/BitCell15 ==
  D : Inport
  WE : Inport  Port=2
  CLK : Inport  Port=3
  Constant : Constant
  D Flip-Flop : simulink_extras/Flip Flops/D Flip-Flop
  Logical Operator : Logic  Operator=NOT  IconShape=distinctive  AllPortsSameDT=off  OutDataTypeStr=boolean
  Logical Operator1 : Logic  IconShape=distinctive  AllPortsSameDT=off  OutDataTypeStr=boolean
  Logical Operator2 : Logic  IconShape=distinctive  AllPortsSameDT=off  OutDataTypeStr=boolean
  Logical Operator3 : Logic  Operator=OR  IconShape=distinctive  AllPortsSameDT=off  OutDataTypeStr=boolean
  Q : Outport
  wires:
  Logical Operator2/1 -> Logical Operator3/2
  CLK/1 -> D Flip-Flop/2
  Logical Operator1/1 -> Logical Operator3/1
  Constant/1 -> D Flip-Flop/3
  D Flip-Flop/1 -> Q/1, Logical Operator2/2
  Logical Operator3/1 -> D Flip-Flop/1
  Logical Operator/1 -> Logical Operator2/1
  WE/1 -> Logical Operator/1, Logical Operator1/2
  D/1 -> Logical Operator1/1

== system Digital-Memory-Architecture/BitCell16 ==
  D : Inport
  WE : Inport  Port=2
  CLK : Inport  Port=3
  Constant : Constant
  D Flip-Flop : simulink_extras/Flip Flops/D Flip-Flop
  Logical Operator : Logic  Operator=NOT  IconShape=distinctive  AllPortsSameDT=off  OutDataTypeStr=boolean
  Logical Operator1 : Logic  IconShape=distinctive  AllPortsSameDT=off  OutDataTypeStr=boolean
  Logical Operator2 : Logic  IconShape=distinctive  AllPortsSameDT=off  OutDataTypeStr=boolean
  Logical Operator3 : Logic  Operator=OR  IconShape=distinctive  AllPortsSameDT=off  OutDataTypeStr=boolean
  Q : Outport
  wires:
  Logical Operator2/1 -> Logical Operator3/2
  CLK/1 -> D Flip-Flop/2
  Logical Operator1/1 -> Logical Operator3/1
  Constant/1 -> D Flip-Flop/3
  D Flip-Flop/1 -> Q/1, Logical Operator2/2
  Logical Operator3/1 -> D Flip-Flop/1
  Logical Operator/1 -> Logical Operator2/1
  WE/1 -> Logical Operator/1, Logical Operator1/2
  D/1 -> Logical Operator1/1

== system Digital-Memory-Architecture/BitCell17 ==
  D : Inport
  WE : Inport  Port=2
  CLK : Inport  Port=3
  Constant : Constant
  D Flip-Flop : simulink_extras/Flip Flops/D Flip-Flop
  Logical Operator : Logic  Operator=NOT  IconShape=distinctive  AllPortsSameDT=off  OutDataTypeStr=boolean
  Logical Operator1 : Logic  IconShape=distinctive  AllPortsSameDT=off  OutDataTypeStr=boolean
  Logical Operator2 : Logic  IconShape=distinctive  AllPortsSameDT=off  OutDataTypeStr=boolean
  Logical Operator3 : Logic  Operator=OR  IconShape=distinctive  AllPortsSameDT=off  OutDataTypeStr=boolean
  Q : Outport
  wires:
  Logical Operator2/1 -> Logical Operator3/2
  CLK/1 -> D Flip-Flop/2
  Logical Operator1/1 -> Logical Operator3/1
  Constant/1 -> D Flip-Flop/3
  D Flip-Flop/1 -> Q/1, Logical Operator2/2
  Logical Operator3/1 -> D Flip-Flop/1
  Logical Operator/1 -> Logical Operator2/1
  WE/1 -> Logical Operator/1, Logical Operator1/2
  D/1 -> Logical Operator1/1

== system Digital-Memory-Architecture/BitCell18 ==
  D : Inport
  WE : Inport  Port=2
  CLK : Inport  Port=3
  Constant : Constant
  D Flip-Flop : simulink_extras/Flip Flops/D Flip-Flop
  Logical Operator : Logic  Operator=NOT  IconShape=distinctive  AllPortsSameDT=off  OutDataTypeStr=boolean
  Logical Operator1 : Logic  IconShape=distinctive  AllPortsSameDT=off  OutDataTypeStr=boolean
  Logical Operator2 : Logic  IconShape=distinctive  AllPortsSameDT=off  OutDataTypeStr=boolean
  Logical Operator3 : Logic  Operator=OR  IconShape=distinctive  AllPortsSameDT=off  OutDataTypeStr=boolean
  Q : Outport
  wires:
  Logical Operator2/1 -> Logical Operator3/2
  CLK/1 -> D Flip-Flop/2
  Logical Operator1/1 -> Logical Operator3/1
  Constant/1 -> D Flip-Flop/3
  D Flip-Flop/1 -> Q/1, Logical Operator2/2
  Logical Operator3/1 -> D Flip-Flop/1
  Logical Operator/1 -> Logical Operator2/1
  WE/1 -> Logical Operator/1, Logical Operator1/2
  D/1 -> Logical Operator1/1

== system Digital-Memory-Architecture/BitCell19 ==
  D : Inport
  WE : Inport  Port=2
  CLK : Inport  Port=3
  Constant : Constant
  D Flip-Flop : simulink_extras/Flip Flops/D Flip-Flop
  Logical Operator : Logic  Operator=NOT  IconShape=distinctive  AllPortsSameDT=off  OutDataTypeStr=boolean
  Logical Operator1 : Logic  IconShape=distinctive  AllPortsSameDT=off  OutDataTypeStr=boolean
  Logical Operator2 : Logic  IconShape=distinctive  AllPortsSameDT=off  OutDataTypeStr=boolean
  Logical Operator3 : Logic  Operator=OR  IconShape=distinctive  AllPortsSameDT=off  OutDataTypeStr=boolean
  Q : Outport
  wires:
  Logical Operator2/1 -> Logical Operator3/2
  CLK/1 -> D Flip-Flop/2
  Logical Operator1/1 -> Logical Operator3/1
  Constant/1 -> D Flip-Flop/3
  D Flip-Flop/1 -> Q/1, Logical Operator2/2
  Logical Operator3/1 -> D Flip-Flop/1
  Logical Operator/1 -> Logical Operator2/1
  WE/1 -> Logical Operator/1, Logical Operator1/2
  D/1 -> Logical Operator1/1

== system Digital-Memory-Architecture/BitCell2 ==
  D : Inport
  WE : Inport  Port=2
  CLK : Inport  Port=3
  Constant : Constant
  D Flip-Flop : simulink_extras/Flip Flops/D Flip-Flop
  Logical Operator : Logic  Operator=NOT  IconShape=distinctive  AllPortsSameDT=off  OutDataTypeStr=boolean
  Logical Operator1 : Logic  IconShape=distinctive  AllPortsSameDT=off  OutDataTypeStr=boolean
  Logical Operator2 : Logic  IconShape=distinctive  AllPortsSameDT=off  OutDataTypeStr=boolean
  Logical Operator3 : Logic  Operator=OR  IconShape=distinctive  AllPortsSameDT=off  OutDataTypeStr=boolean
  Q : Outport
  wires:
  Logical Operator2/1 -> Logical Operator3/2
  CLK/1 -> D Flip-Flop/2
  Logical Operator1/1 -> Logical Operator3/1
  Constant/1 -> D Flip-Flop/3
  D Flip-Flop/1 -> Q/1, Logical Operator2/2
  Logical Operator3/1 -> D Flip-Flop/1
  Logical Operator/1 -> Logical Operator2/1
  WE/1 -> Logical Operator/1, Logical Operator1/2
  D/1 -> Logical Operator1/1

== system Digital-Memory-Architecture/BitCell20 ==
  D : Inport
  WE : Inport  Port=2
  CLK : Inport  Port=3
  Constant : Constant
  D Flip-Flop : simulink_extras/Flip Flops/D Flip-Flop
  Logical Operator : Logic  Operator=NOT  IconShape=distinctive  AllPortsSameDT=off  OutDataTypeStr=boolean
  Logical Operator1 : Logic  IconShape=distinctive  AllPortsSameDT=off  OutDataTypeStr=boolean
  Logical Operator2 : Logic  IconShape=distinctive  AllPortsSameDT=off  OutDataTypeStr=boolean
  Logical Operator3 : Logic  Operator=OR  IconShape=distinctive  AllPortsSameDT=off  OutDataTypeStr=boolean
  Q : Outport
  wires:
  Logical Operator2/1 -> Logical Operator3/2
  CLK/1 -> D Flip-Flop/2
  Logical Operator1/1 -> Logical Operator3/1
  Constant/1 -> D Flip-Flop/3
  D Flip-Flop/1 -> Q/1, Logical Operator2/2
  Logical Operator3/1 -> D Flip-Flop/1
  Logical Operator/1 -> Logical Operator2/1
  WE/1 -> Logical Operator/1, Logical Operator1/2
  D/1 -> Logical Operator1/1

== system Digital-Memory-Architecture/BitCell21 ==
  D : Inport
  WE : Inport  Port=2
  CLK : Inport  Port=3
  Constant : Constant
  D Flip-Flop : simulink_extras/Flip Flops/D Flip-Flop
  Logical Operator : Logic  Operator=NOT  IconShape=distinctive  AllPortsSameDT=off  OutDataTypeStr=boolean
  Logical Operator1 : Logic  IconShape=distinctive  AllPortsSameDT=off  OutDataTypeStr=boolean
  Logical Operator2 : Logic  IconShape=distinctive  AllPortsSameDT=off  OutDataTypeStr=boolean
  Logical Operator3 : Logic  Operator=OR  IconShape=distinctive  AllPortsSameDT=off  OutDataTypeStr=boolean
  Q : Outport
  wires:
  Logical Operator2/1 -> Logical Operator3/2
  CLK/1 -> D Flip-Flop/2
  Logical Operator1/1 -> Logical Operator3/1
  Constant/1 -> D Flip-Flop/3
  D Flip-Flop/1 -> Q/1, Logical Operator2/2
  Logical Operator3/1 -> D Flip-Flop/1
  Logical Operator/1 -> Logical Operator2/1
  WE/1 -> Logical Operator/1, Logical Operator1/2
  D/1 -> Logical Operator1/1

== system Digital-Memory-Architecture/BitCell22 ==
  D : Inport
  WE : Inport  Port=2
  CLK : Inport  Port=3
  Constant : Constant
  D Flip-Flop : simulink_extras/Flip Flops/D Flip-Flop
  Logical Operator : Logic  Operator=NOT  IconShape=distinctive  AllPortsSameDT=off  OutDataTypeStr=boolean
  Logical Operator1 : Logic  IconShape=distinctive  AllPortsSameDT=off  OutDataTypeStr=boolean
  Logical Operator2 : Logic  IconShape=distinctive  AllPortsSameDT=off  OutDataTypeStr=boolean
  Logical Operator3 : Logic  Operator=OR  IconShape=distinctive  AllPortsSameDT=off  OutDataTypeStr=boolean
  Q : Outport
  wires:
  Logical Operator2/1 -> Logical Operator3/2
  CLK/1 -> D Flip-Flop/2
  Logical Operator1/1 -> Logical Operator3/1
  Constant/1 -> D Flip-Flop/3
  D Flip-Flop/1 -> Q/1, Logical Operator2/2
  Logical Operator3/1 -> D Flip-Flop/1
  Logical Operator/1 -> Logical Operator2/1
  WE/1 -> Logical Operator/1, Logical Operator1/2
  D/1 -> Logical Operator1/1
